simulink model "pid_motor_sys"  (R2017b)
settings: Solver=VariableStepAuto  StartTime=0.0  StopTime=1  RelTol=1e-3
InitFcn:
  | before_simulation
values from neighbouring files (symbols this model uses):
  J = 0.08    [before_simulation.m]
  Kb = 0.87    [before_simulation.m]
  Kf = 0.043    [before_simulation.m]
  Km = 1.34    [before_simulation.m]
  L = 0.05    [before_simulation.m]
  R = 1.7    [before_simulation.m]
libraries: simulink_extras x4, simulink x2
settings Model: Creator=Iman  LastModifiedBy=Iman

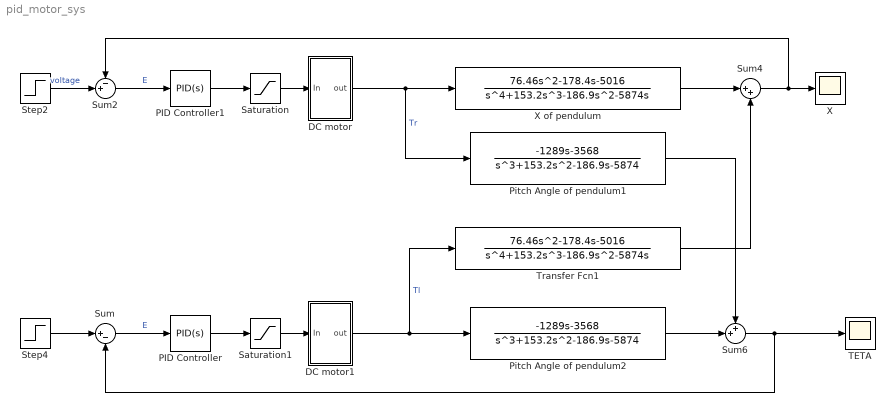
== system pid_motor_sys ==
  DC motor : Subsystem
  DC motor1 : Subsystem
  PID Controller : simulink/Continuous/PID Controller  Controller=PID  TimeDomain=Continuous-time  SampleTime=-1  IntegratorMethod=Forward Euler  FilterMethod=Forward Euler  Form=Parallel  UseFilter=on  ControllerParametersSource=internal  P=-5.4  I=-57.6  D=-0.1224  N=7424.97395554025  InitialConditionSource=internal  InitialConditionForIntegrator=0  InitialConditionForFilter=0  ExternalReset=none  LimitOutput=off  UpperSaturationLimit=inf  LowerSaturationLimit=-inf  LinearizeAsGain=on  AntiWindupMode=none  Kb=1  TrackingMode=off  Kt=1  PParamMin=[]  PParamMax=[]  IParamMin=[]  IParamMax=[]  DParamMin=[]  DParamMax=[]  NParamMin=[]  NParamMax=[]  KbParamMin=[]  KbParamMax=[]  KtParamMin=[]  KtParamMax=[]  POutMin=[]  POutMax=[]  IOutMin=[]  IOutMax=[]  DOutMin=[]  DOutMax=[]  NOutMin=[]  NOutMax=[]  KbOutMin=[]  KbOutMax=[]  KtOutMin=[]  KtOutMax=[]  IntegratorOutMin=[]  IntegratorOutMax=[]  FilterOutMin=[]  FilterOutMax=[]  SumOutMin=[]  SumOutMax=[]  SumI1OutMin=[]  SumI1OutMax=[]  SumI2OutMin=[]  SumI2OutMax=[]  SumI3OutMin=[]  SumI3OutMax=[]  SumDOutMin=[]  SumDOutMax=[]  SaturationOutMin=[]  SaturationOutMax=[]  IntegratorContinuousStateAttributes=''  IntegratorStateMustResolveToSignalObject=off  IntegratorRTWStateStorageClass=Auto  FilterContinuousStateAttributes=''  FilterStateMustResolveToSignalObject=off  FilterRTWStateStorageClass=Auto  DifferentiatorICPrevScaledInput=0  DifferentiatorOutMin=[]  DifferentiatorOutMax=[]  InitialConditionSetting=State (most efficient)  FilterDiffOutCoefMin=[]  FilterDiffOutCoefMax=[]  SumDenOutMin=[]  SumDenOutMax=[]  SumNumOutMin=[]  SumNumOutMax=[]  ReciprocalOutMin=[]  ReciprocalOutMax=[]  DivideOutMin=[]  DivideOutMax=[]  TunerSelectOption=Transfer Function Based (PID Tuner App)
  PID Controller1 : simulink/Continuous/PID Controller  Controller=PID  TimeDomain=Continuous-time  SampleTime=-1  IntegratorMethod=Forward Euler  FilterMethod=Forward Euler  Form=Parallel  UseFilter=on  ControllerParametersSource=internal  P=-10  I=-50  D=-0.2  N=3892.86009234078  InitialConditionSource=internal  InitialConditionForIntegrator=0  InitialConditionForFilter=0  ExternalReset=none  LimitOutput=off  UpperSaturationLimit=inf  LowerSaturationLimit=-inf  LinearizeAsGain=on  AntiWindupMode=none  Kb=1  TrackingMode=off  Kt=1  PParamMin=[]  PParamMax=[]  IParamMin=[]  IParamMax=[]  DParamMin=[]  DParamMax=[]  NParamMin=[]  NParamMax=[]  KbParamMin=[]  KbParamMax=[]  KtParamMin=[]  KtParamMax=[]  POutMin=[]  POutMax=[]  IOutMin=[]  IOutMax=[]  DOutMin=[]  DOutMax=[]  NOutMin=[]  NOutMax=[]  KbOutMin=[]  KbOutMax=[]  KtOutMin=[]  KtOutMax=[]  IntegratorOutMin=[]  IntegratorOutMax=[]  FilterOutMin=[]  FilterOutMax=[]  SumOutMin=[]  SumOutMax=[]  SumI1OutMin=[]  SumI1OutMax=[]  SumI2OutMin=[]  SumI2OutMax=[]  SumI3OutMin=[]  SumI3OutMax=[]  SumDOutMin=[]  SumDOutMax=[]  SaturationOutMin=[]  SaturationOutMax=[]  IntegratorContinuousStateAttributes=''  IntegratorStateMustResolveToSignalObject=off  IntegratorRTWStateStorageClass=Auto  FilterContinuousStateAttributes=''  FilterStateMustResolveToSignalObject=off  FilterRTWStateStorageClass=Auto  DifferentiatorICPrevScaledInput=0  DifferentiatorOutMin=[]  DifferentiatorOutMax=[]  InitialConditionSetting=State (most efficient)  FilterDiffOutCoefMin=[]  FilterDiffOutCoefMax=[]  SumDenOutMin=[]  SumDenOutMax=[]  SumNumOutMin=[]  SumNumOutMax=[]  ReciprocalOutMin=[]  ReciprocalOutMax=[]  DivideOutMin=[]  DivideOutMax=[]  TunerSelectOption=Transfer Function Based (PID Tuner App)
  Pitch Angle of pendulum1 : TransferFcn  Numerator="[-1289  -3568]"  Denominator="[1 153.2  -186.9  -5874]"  ContinuousStateAttributes='TETA'
  Pitch Angle of pendulum2 : TransferFcn  Numerator="[-1289  -3568]"  Denominator="[1 153.2  -186.9  -5874]"  ContinuousStateAttributes='TETA'
  Saturation : Saturate  UpperLimit=12  LowerLimit=-12
  Saturation1 : Saturate  UpperLimit=12  LowerLimit=-12
  Step2 : Step  Time=0  SampleTime=0.1
  Step4 : Step  Time=0  After=0  SampleTime=0.1
  Sum : Sum  Inputs=|+-
  Sum2 : Sum  Inputs=-+|
  Sum4 : Sum  Inputs=|++
  Sum6 : Sum  Inputs=++|
  TETA : Scope
  Transfer Fcn1 : TransferFcn  Numerator=[76.46 -178.4 -5016]  Denominator="[1 153.2  -186.9  -5874  0]"
  X : Scope
  X of pendulum : TransferFcn  Numerator=[76.46 -178.4 -5016]  Denominator="[1 153.2  -186.9  -5874  0]"
  wires:
  Sum6/1 -> Sum/2, TETA/1
  Sum2/1 -> PID Controller1/1  "E"
  Step4/1 -> Sum/1
  Transfer Fcn1/1 -> Sum4/2
  Sum4/1 -> Sum2/1, X/1
  Sum/1 -> PID Controller/1  "E"
  X of pendulum/1 -> Sum4/1
  DC motor/1(out) -> Pitch Angle of pendulum1/1, X of pendulum/1  "Tr"
  DC motor1/1(out) -> Pitch Angle of pendulum2/1, Transfer Fcn1/1  "Tl"
  Pitch Angle of pendulum2/1 -> Sum6/2
  Pitch Angle of pendulum1/1 -> Sum6/1
  Step2/1 -> Sum2/2  "voltage"
  Saturation/1 -> DC motor/1(In)
  PID Controller1/1 -> Saturation/1
  PID Controller/1 -> Saturation1/1
  Saturation1/1 -> DC motor1/1(In)

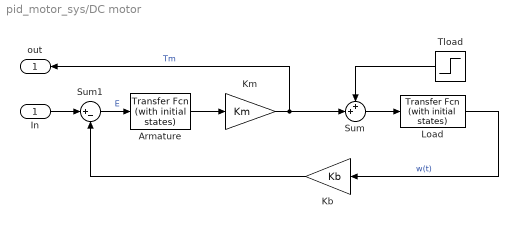
== system pid_motor_sys/DC motor ==
  In : Inport
  Armature : simulink_extras/Additional Linear/Transfer Fcn (with initial states)  N=[1]  D=[L R]  X0=0
  Kb : Gain  Gain=Kb
  Km : Gain  Gain=Km
  Load : simulink_extras/Additional Linear/Transfer Fcn (with initial states)  N=[1]  D=[J Kf]  X0=0
  Sum : Sum  Inputs=++|
  Sum1 : Sum  Inputs=|+-
  Tload : Step  Time=0.2  After=0  SampleTime=0
  out : Outport
  wires:
  Load/1 -> Kb/1  "w(t)"
  In/1 -> Sum1/1
  Tload/1 -> Sum/1
  Armature/1 -> Km/1
  Sum/1 -> Load/1
  Kb/1 -> Sum1/2
  Sum1/1 -> Armature/1  "E"
  Km/1 -> Sum/2, out/1  "Tm"

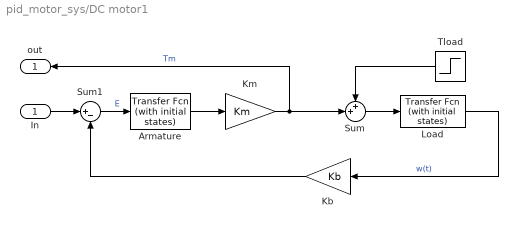
== system pid_motor_sys/DC motor1 ==
  In : Inport
  Armature : simulink_extras/Additional Linear/Transfer Fcn (with initial states)  N=[1]  D=[L R]  X0=0
  Kb : Gain  Gain=Kb
  Km : Gain  Gain=Km
  Load : simulink_extras/Additional Linear/Transfer Fcn (with initial states)  N=[1]  D=[J Kf]  X0=0
  Sum : Sum  Inputs=++|
  Sum1 : Sum  Inputs=|+-
  Tload : Step  Time=0.2  After=0  SampleTime=0
  out : Outport
  wires:
  Load/1 -> Kb/1  "w(t)"
  In/1 -> Sum1/1
  Tload/1 -> Sum/1
  Armature/1 -> Km/1
  Sum/1 -> Load/1
  Kb/1 -> Sum1/2
  Sum1/1 -> Armature/1  "E"
  Km/1 -> Sum/2, out/1  "Tm"
